simulink model "Seal"  (R2025a)
settings: Solver=FixedStepDiscrete  StartTime=0.0  StopTime=30  FixedStep=0.025  RelTol=1e-3
model workspace (MATLAB code in the model file + MAT data in the model file):
  | cmdLim = Simulink.Parameter;
  | cmdLim.Value = 15;
  | cmdLim.Description = 'Limit for controlling the maximum surface command angle.';
  | cmdLim.Min = 0;
  | cmdLim.Max = 90;
  | cmdLim.DocUnits = 'deg';
  | 
  | dispGain = Simulink.Parameter;
  | dispGain.Value = 0.75;
  | dispGain.Description = 'Gain applied to the displacement error.';
  | dispGain.Min = 0;
  | dispGain.Max = [];
  | dispGain.DocUnits = 'deg/sec/deg';
  | 
  | dispLim = Simulink.Parameter;
  | dispLim.Value = 30;
  | dispLim.Description = 'Limit for controlling the maximum commanded angle.';
  | dispLim.Min = 0;
  | dispLim.Max = 180;
  | dispLim.DocUnits = 'deg';
  | 
  | intGain = Simulink.Parameter;
  | intGain.Value = 0.5;
  | intGain.Description = 'Gain applied to the integral error.';
  | intGain.Min = 0;
  | intGain.Max = [];
  | intGain.DocUnits = 'deg/sec/deg/sec';
  | 
  | intLim = Simulink.Parameter;
  | intLim.Value = 5;
  | intLim.Description = 'Limit for controlling the maximum commanded angle.';
  | intLim.Min = 0;
  | intLim.Max = 90;
  | intLim.DocUnits = 'deg';
  | 
  | rateGain = Simulink.Parameter;
  | rateGain.Value = 2;
  | rateGain.Description = 'Gain applied to the rate error.';
  | rateGain.Min = 0;
  | rateGain.Max = [];
  | rateGain.DocUnits = 'deg/deg/sec';
  | 
  | rateLim = Simulink.Parameter;
  | rateLim.Value = 6;
  | rateLim.Description = 'Limit for controlling the maximum commanded angle.';
  | rateLim.Min = 0;
  | rateLim.Max = 180;
  | rateLim.DocUnits = 'deg/sec';
  | 
  | hdgGain = Simulink.Parameter;
  | hdgGain.Value = 0.015;
undefined symbols (not defined in the file or in its folder): CurrentCommand, KiSpeed, Kp, KpSpeed, PositionCommand, SpeedCommand
libraries: simulink x1
Description:
  | This model represents a basic roll axis autopilot with two operating
  | modes; roll attitude hold and heading hold. The mode logic for these
  | modes is external to this model.  The model architecture represents the
  | heading hold mode and basic roll attitude function as referenced models.
  | 
  | The roll attitude control function is a PID controller that uses roll
  | attitude and roll rate feedback to produce an aileron command.  The
  | input to the controller will be either a basic roll angle reference or a
  | roll command to track the desired heading.
settings Model: RequirementInfo={} %GIDa_fe9045fd_0412_4b6e_8206_617cc20e6fde  DataDictionary=SEALGenericTypes_1.sldd  FPTRunName=Active  ModifiedByFormat=The MathWorks, Inc.  Creator=The MathWorks, Inc.  LastModifiedBy=The MathWorks, Inc.
settings SolverCC: AlgebraicLoopSolver=TrustRegion
settings DataIOCC: ExternalInput=xin  SaveFormat=StructureWithTime  SaveOutput=off  SignalLogging=off  DSMLogging=off  SaveTime=off  ReturnWorkspaceOutputs=off
settings OptimizationCC: DefaultParameterBehavior=Inlined  UseDivisionForNetSlopeComputation=on  UseFloatMulNetSlope=on  InlineInvariantSignals=on  ReuseModelBlockBuffer=off  EnhancedBackFolding=on  BooleansAsBitfields=on  PassReuseOutputArgsAs=Individual arguments  ExpressionDepthLimit=2147483647.0  StateBitsets=on  DataBitsets=on  ZeroExternalMemoryAtStartup=off  ZeroInternalMemoryAtStartup=off  NoFixptDivByZeroProtection=on  EfficientFloat2IntCast=on  LifeSpan=inf  MaxStackSize=inf  EfficientTunableParamExpr=on
settings DebuggingCC: SignalRangeChecking=error  ReadBeforeWriteMsg=EnableAllAsError  WriteAfterWriteMsg=EnableAllAsError  WriteAfterReadMsg=EnableAllAsError  AlgebraicLoopMsg=error  ArtificialAlgebraicLoopMsg=error  SaveWithDisabledLinksMsg=error  SaveWithParameterizedLinksMsg=error  CheckExecutionContextPreStartOutputMsg=on  BlockPriorityViolationMsg=error  MaxConsecutiveZCsMsg=warning  SolverPrmCheckMsg=error  InheritedTsInSrcMsg=error  SingleTaskRateTransMsg=error  TasksWithSamePriorityMsg=error  SigSpecEnsureSampleTimeMsg=error  IntegerOverflowMsg=error  ParameterUnderflowMsg=error  ParameterPrecisionLossMsg=none  ParameterTunabilityLossMsg=error  UnderSpecifiedDataTypeMsg=error  UnnecessaryDatatypeConvMsg=warning  VectorMatrixConversionMsg=error  SignalLabelMismatchMsg=error  UnconnectedInputMsg=error  UnconnectedOutputMsg=error  UnconnectedLineMsg=error  SFcnCompatibilityMsg=error  UniqueDataStoreMsg=error  BusObjectLabelMismatch=error  RootOutportRequireBusObject=error  AssertControl=DisableAll  AllowSymbolicDim=off  ModelReferenceIOMismatchMessage=error  UnknownTsInhSupMsg=error  ModelReferenceDataLoggingMessage=error  ModelReferenceSymbolNameMessage=none  StateNameClashWarn=warning  StrictBusMsg=ErrorOnBusTreatedAsVector  NonBusSignalsTreatedAsBus=error  SFInvalidInputDataAccessInChartInitDiag=error  SFTransitionOutsideNaturalParentDiag=error  SFUnreachableExecutionPathDiag=error  SFUndirectedBroadcastEventsDiag=error  SFExecutionAtInitializationDiag=none  IntegerSaturationMsg=error  ArithmeticOperatorsInVariantConditions=warning
settings HardwareCC: ProdBitPerChar=16.0  ProdBitPerInt=16.0  ProdBitPerPointer=32.0  ProdBitPerSizeT=32.0  ProdBitPerPtrDiffT=32.0  ProdLargestAtomicInteger=Integer  ProdLargestAtomicFloat=None  ProdWordSize=16.0  ProdHWDeviceType=Texas Instruments->C2000  TargetHWDeviceType=32-bit Generic
settings ModelReferenceCC: EnableRefExpFcnMdlSchedulingChecks=on  ModelReferenceNumInstancesAllowed=Single  PropagateSignalLabelsOutOfModel=off
settings SFSimCC: SimUseLocalCustomCode=off  MATLABDynamicMemAlloc=off
settings SFSimCC: SimCustomHeaderCode=|
  | #include "CANServer.h"
  | #include "DeviceSetup.h"
settings SFSimCC: SimUserSources=|
  | .\ExternalCode\CANServer.c
  | .\ExternalCode\DeviceSetup.c
settings RTWCC: SystemTargetFile=ert.tlc  GenCodeOnly=on  TemplateMakefile=ert_default_tmf  PostCodeGenCommand=PrepWrapper  GenerateReport=on  RTWVerbose=off  RTWUseLocalCustomCode=off  RTWUseSimCustomCode=on  BuildConfiguration=Faster Runs  IncludeHyperlinkInReport=on  LaunchReport=on  GenerateTraceInfo=on  GenerateTraceReport=on  GenerateTraceReportSl=on  GenerateTraceReportSf=on  GenerateTraceReportEml=on  GenerateCodeMetricsReport=on  GPUComputeCapability=3.5  DLArmComputeVersion=19.05  Description=Embedded Coder
settings RTWCC: CustomHeaderCode=|
  | #include "CANServer.h"
  | #include "DeviceSetup.h"
settings RTWCC: CustomSource=|
  | .\ExternalCode\CANServer.c
  | .\ExternalCode\DeviceSetup.c
settings CodeAppCC: ForceParamTrailComments=on  IgnoreCustomStorageClasses=off  SimulinkDataObjDesc=on  CustomSymbolStrGlobalVar=rt$N$M  CustomSymbolStrType=$N$M  CustomSymbolStrFcn=$N$M$F  CustomSymbolStrMacro=$N$M  InsertBlockDesc=on  ReqsInCode=on
settings ERTTargetCC: ExtModeTransport=0.0  ExtModeStaticAlloc=off  ExtModeMexFile=ext_comm  ExtModeIntrfLevel=Level1  ERTCustomFileTemplate=example_file_process.tlc  ERTFilePackagingFormat=CompactWithDataFile  ConvertIfToSwitch=off  SuppressUnreachableDefaultCases=off  DynamicArrayContainerType=coder::array  UtilityFuncGeneration=Shared location  MultiwordLength=2048.0  GenerateSampleERTMain=on  IncludeMdlTerminateFcn=off  CombineSignalStateStructs=on  SuppressErrorStatus=on  SupportAbsoluteTime=off  SubcomponentCodeInterfacePackaging=Nonreusable function  SupportNonFinite=off  SupportComplex=off
settings ConfigComp: CovScope=ReferencedModels  CovSaveName=covdata_rollAP  CovMetricSettings=dcmtrwe  CovHTMLOptions=-sRT=1 -aTS=1 -bRG=1 -bTC=1 -hTR=1 -nFC=0 -scm=1 -bcm=1 -xEv=0  CovSaveCumulativeToWorkspaceVar=on  CovSaveSingleToWorkspaceVar=on  CovCumulativeVarName=covCumulativeData_rollAP  CovReportOnPause=off  CovExternalEMLEnable=off  CovSFcnEnable=off  DVMaxProcessTime=300.0  DVModelCoverageObjectives=MCDC  DVMaxTestCaseSteps=500.0  DVTestSuiteOptimization=Auto  DVAbsoluteTolerance=1.0e-5  DVDefectChecker=off  DVDetectActiveLogic=on  DVMaxViolationSteps=20.0  DVSaveHarnessModel=on  DVModelReferenceHarness=on  DVHarnessSource=Signal Editor  DVSaveReport=on  DVRebuildModelRepresentation=Always  DVActiveTab=0.0

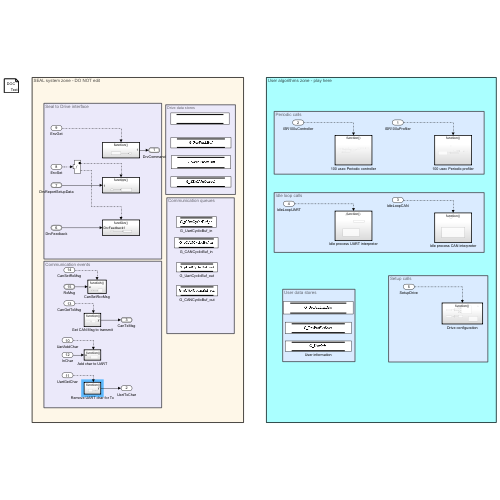
[thumbnail: Simulink's stored preview of the top-level diagram]
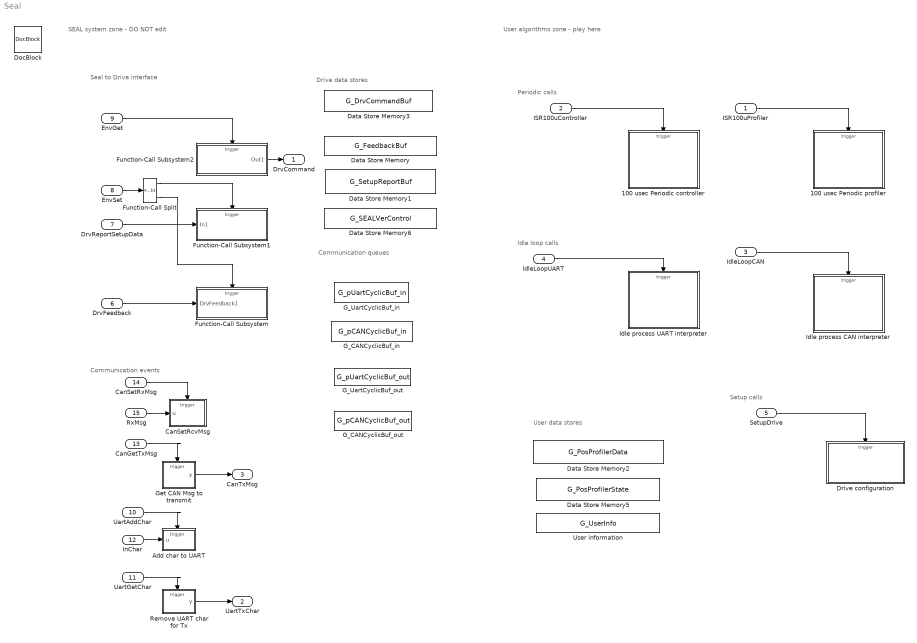
== system Seal ==
  note: User algorithms zone - play here
  note: SEAL system zone - DO NOT edit
  note: Communication queues
  note: Communication events
  note: Seal to Drive interface
  note: Setup calls
  note: Idle loop calls
  note: Periodic calls
  note: User data stores
  note: Drive data stores
  ISR100uProfiler : Inport  Priority=1  OutputFunctionCall=on
  ISR100uController : Inport  Priority=1  Port=2  OutputFunctionCall=on
  IdleLoopCAN : Inport  Priority=1  Port=3  OutputFunctionCall=on
  IdleLoopUART : Inport  Priority=1  Port=4  OutputFunctionCall=on
  SetupDrive : Inport  Priority=1  Port=5  OutputFunctionCall=on
  DrvFeedback : Inport  Port=6  OutDataTypeStr=Bus: FeedbackBuf_T  PortDimensions=1  BusOutputAsStruct=on
  DrvReportSetupData : Inport  Port=7  OutDataTypeStr=Bus: SetupReportBuf_T  PortDimensions=1  BusOutputAsStruct=on
  EnvSet : Inport  Priority=1  Port=8  OutputFunctionCall=on
  EnvGet : Inport  Priority=1  Port=9  OutputFunctionCall=on
  UartAddChar : Inport  Priority=1  Port=10  OutputFunctionCall=on
  UartGetChar : Inport  Priority=1  Port=11  OutputFunctionCall=on
  InChar : Inport  Port=12  PortDimensions=1
  CanGetTxMsg : Inport  Priority=1  Port=13  OutputFunctionCall=on
  CanSetRxMsg : Inport  Priority=1  Port=14  OutputFunctionCall=on
  RxMsg : Inport  Port=15  OutDataTypeStr=Bus: CANMessage_T  PortDimensions=1  BusOutputAsStruct=on
  100 usec Periodic controller : Subsystem  TreatAsAtomicUnit=on
  100 usec Periodic profiler : Subsystem  TreatAsAtomicUnit=on
  Add char to UART : Subsystem  TreatAsAtomicUnit=on
  CanSetRcvMsg : Subsystem  TreatAsAtomicUnit=on
  Data Store Memory : DataStoreMemory  DataStoreName=G_FeedbackBuf  WriteAfterWriteMsg=warning  VectorParams1D=off  ShowAdditionalParam=off  OutDataTypeStr=Bus: FeedbackBuf_T  StateMustResolveToSignalObject=on
  Data Store Memory1 : DataStoreMemory  DataStoreName=G_SetupReportBuf  WriteAfterWriteMsg=warning  ShowAdditionalParam=off  OutDataTypeStr=Bus: SetupReportBuf_T  StateMustResolveToSignalObject=on
  Data Store Memory2 : DataStoreMemory  DataStoreName=G_PosProfilerData  WriteAfterWriteMsg=warning  InitialValue=PosProfilerData_init  ShowAdditionalParam=off  OutDataTypeStr=Bus: PosProfilerData_T
  Data Store Memory3 : DataStoreMemory  DataStoreName=G_DrvCommandBuf  WriteAfterWriteMsg=warning  ShowAdditionalParam=off  OutDataTypeStr=Bus: DrvCommandBuf_T  StateMustResolveToSignalObject=on
  Data Store Memory5 : DataStoreMemory  DataStoreName=G_PosProfilerState  WriteAfterWriteMsg=warning  InitialValue=PosProfilerState_init  ShowAdditionalParam=off  OutDataTypeStr=Bus: PosProfilerState_T
  Data Store Memory6 : DataStoreMemory  DataStoreName=G_SEALVerControl  WriteAfterWriteMsg=warning  InitialValue=SEALVerControl_init  ShowAdditionalParam=off  OutDataTypeStr=Bus: SEALVerControl_T  StateMustResolveToSignalObject=on
  DocBlock : simulink/Model-Wide Utilities/DocBlock  DocumentType=Text
      content=|
      | These are the global variables for communication with the hosting servo drive.
      | NEVER remove them!
      | They are declared as global variables of the drive.
      | Their structure   is given in the p-coded file HostDriveInterface.p
      |
      | G_DrvCommandBuf     stores the commands to the servo drive.
      | G_SetupReportBuf    reports the setup parameters of the hosting servo drive to the SEAL application
      | FeedbackBuf         reports the feedback and sensor values to the SEAL application.
  Drive configuration : Subsystem  TreatAsAtomicUnit=on
  Function-Call Split : FunctionCallSplit  IconShape=distinctive  NumOutputPorts=2  OutputPortLayout=default
  Function-Call Subsystem : Subsystem  TreatAsAtomicUnit=on
  Function-Call Subsystem1 : Subsystem  TreatAsAtomicUnit=on
  Function-Call Subsystem2 : Subsystem  TreatAsAtomicUnit=on
  G_CANCyclicBuf_in : DataStoreMemory  DataStoreName=G_pCANCyclicBuf_in  WriteAfterWriteMsg=warning  ShowAdditionalParam=off  OutDataTypeStr=Bus: CANCyclicBuf_T  StateMustResolveToSignalObject=on
  G_CANCyclicBuf_out : DataStoreMemory  DataStoreName=G_pCANCyclicBuf_out  WriteAfterWriteMsg=warning  ShowAdditionalParam=off  OutDataTypeStr=Bus: CANCyclicBuf_T  StateMustResolveToSignalObject=on
  G_UartCyclicBuf_in : DataStoreMemory  DataStoreName=G_pUartCyclicBuf_in  WriteAfterWriteMsg=warning  ShowAdditionalParam=off  OutDataTypeStr=Bus: UartCyclicBuf_T  Dimensions=1  StateMustResolveToSignalObject=on
  G_UartCyclicBuf_out : DataStoreMemory  DataStoreName=G_pUartCyclicBuf_out  WriteAfterWriteMsg=warning  ShowAdditionalParam=off  OutDataTypeStr=Bus: UartCyclicBuf_T  StateMustResolveToSignalObject=on
  Get CAN Msg to transmit : Subsystem  TreatAsAtomicUnit=on
  Idle process CAN interpreter : Subsystem  TreatAsAtomicUnit=on
  Idle process UART interpreter : Subsystem  TreatAsAtomicUnit=on
  Remove UART char for Tx : Subsystem  TreatAsAtomicUnit=on
  User information : DataStoreMemory  DataStoreName=G_UserInfo  WriteAfterWriteMsg=warning  InitialValue=G_UserInfo_init  ShowAdditionalParam=off  OutDataTypeStr=Bus: UserInfo_T
  DrvCommand : Outport  OutDataTypeStr=Bus: DrvCommandBuf_T
  UartTxChar : Outport  Port=2  OutDataTypeStr=uint16
  CanTxMsg : Outport  Port=3  OutDataTypeStr=Bus: CANMessage_T  PortDimensions=1
  wires:
  ISR100uProfiler/1 -> 100 usec Periodic profiler/Trigger
  IdleLoopCAN/1 -> Idle process CAN interpreter/Trigger
  IdleLoopUART/1 -> Idle process UART interpreter/Trigger
  SetupDrive/1 -> Drive configuration/Trigger
  ISR100uController/1 -> 100 usec Periodic controller/Trigger
  DrvFeedback/1 -> Function-Call Subsystem/1(DrvFeedback1)
  DrvReportSetupData/1 -> Function-Call Subsystem1/1(In1)
  Function-Call Subsystem2/1(Out1) -> DrvCommand/1
  EnvSet/1 -> Function-Call Split/1
  InChar/1 -> Add char to UART/1(u)
  UartAddChar/1 -> Add char to UART/Trigger
  UartGetChar/1 -> Remove UART char for Tx/Trigger
  Remove UART char for Tx/1(y) -> UartTxChar/1
  CanGetTxMsg/1 -> Get CAN Msg to transmit/Trigger
  Get CAN Msg to transmit/1(y) -> CanTxMsg/1
  CanSetRxMsg/1 -> CanSetRcvMsg/Trigger
  RxMsg/1 -> CanSetRcvMsg/1(u)
  Function-Call Split/2 -> Function-Call Subsystem/Trigger
  Function-Call Split/1 -> Function-Call Subsystem1/Trigger
  EnvGet/1 -> Function-Call Subsystem2/Trigger

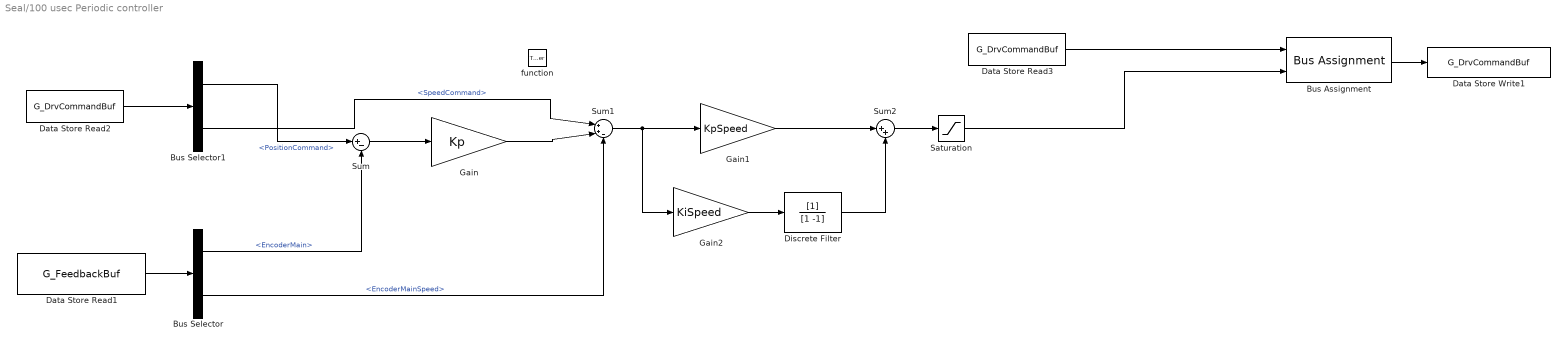
== system Seal/100 usec Periodic controller ==
  function : TriggerPort  TriggerType=function-call  VariantControl=(inherit)
  Bus Assignment : BusAssignment  AssignedSignals=CurrentCommand
  Bus Selector : BusSelector  OutputSignals=EncoderMain,EncoderMainSpeed
  Bus Selector1 : BusSelector  OutputSignals=PositionCommand,SpeedCommand
  Data Store Read1 : DataStoreRead  DataStoreName=G_FeedbackBuf  IndexOptions=Index vector (dialog)  Indices=1  OutputSizes=1
  Data Store Read2 : DataStoreRead  DataStoreName=G_DrvCommandBuf  IndexOptions=Index vector (dialog)  Indices=1  OutputSizes=1
  Data Store Read3 : DataStoreRead  DataStoreName=G_DrvCommandBuf  IndexOptions=Index vector (dialog)  Indices=1  OutputSizes=1
  Data Store Write1 : DataStoreWrite  DataStoreName=G_DrvCommandBuf  IndexOptions=Index vector (dialog)  Indices=1  OutputSizes=1
  Discrete Filter : DiscreteFilter  Denominator=[1 -1]
  Gain : Gain  Gain=Kp
  Gain1 : Gain  Gain=KpSpeed
  Gain2 : Gain  Gain=KiSpeed
  Saturation : Saturate
  Sum : Sum  Inputs=|+-
  Sum1 : Sum  Inputs=|++-
  Sum2 : Sum  Inputs=|++
  wires:
  Data Store Read3/1 -> Bus Assignment/1
  Bus Assignment/1 -> Data Store Write1/1
  Data Store Read1/1 -> Bus Selector/1
  Bus Selector/1 -> Sum/2  "<EncoderMain>"
  Data Store Read2/1 -> Bus Selector1/1
  Bus Selector1/1 -> Sum/1  "<PositionCommand>"
  Sum/1 -> Gain/1
  Gain/1 -> Sum1/2
  Bus Selector1/2 -> Sum1/1  "<SpeedCommand>"
  Bus Selector/2 -> Sum1/3  "<EncoderMainSpeed>"
  Sum1/1 -> Gain2/1, Gain1/1
  Gain2/1 -> Discrete Filter/1
  Gain1/1 -> Sum2/1
  Discrete Filter/1 -> Sum2/2
  Sum2/1 -> Saturation/1
  Saturation/1 -> Bus Assignment/2

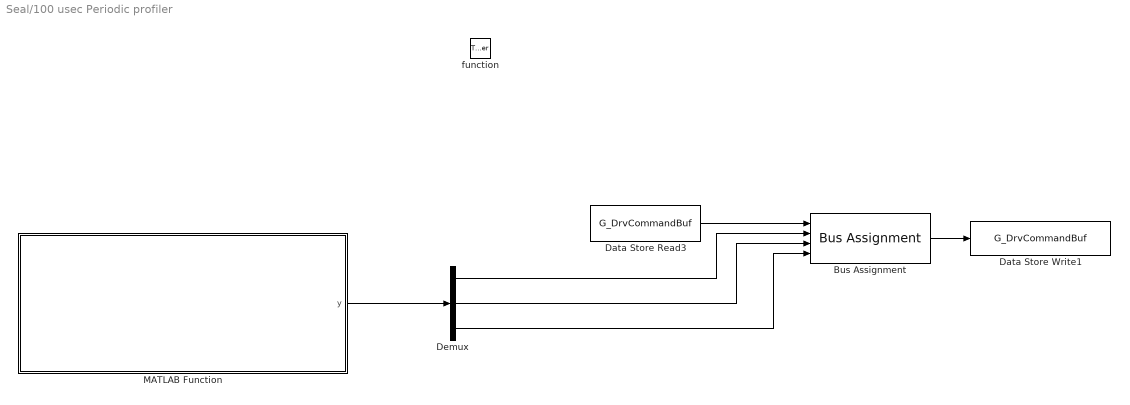
== system Seal/100 usec Periodic profiler ==
  function : TriggerPort  TriggerType=function-call  VariantControl=(inherit)
  Bus Assignment : BusAssignment  AssignedSignals=PositionCommand,SpeedCommand,CurrentCommand
  Data Store Read3 : DataStoreRead  DataStoreName=G_DrvCommandBuf  IndexOptions=Index vector (dialog)  Indices=1  OutputSizes=1
  Data Store Write1 : DataStoreWrite  DataStoreName=G_DrvCommandBuf  IndexOptions=Index vector (dialog)  Indices=1  OutputSizes=1
  Demux : Demux  Outputs=3
  MATLAB Function : MATLAB Function  TreatAsAtomicUnit=on
  wires:
  Data Store Read3/1 -> Bus Assignment/1
  MATLAB Function/1(y) -> Demux/1
  Demux/1 -> Bus Assignment/2
  Demux/2 -> Bus Assignment/3
  Demux/3 -> Bus Assignment/4
  Bus Assignment/1 -> Data Store Write1/1

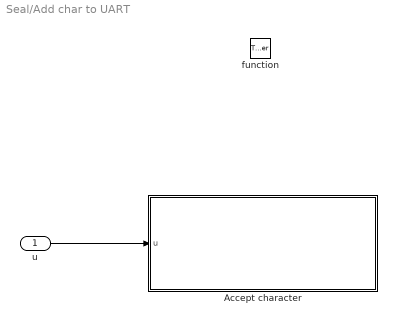
== system Seal/Add char to UART ==
  u : Inport  OutDataTypeStr=uint16  PortDimensions=1
  function : TriggerPort  TriggerType=function-call  VariantControl=(inherit)
  Accept character : MATLAB Function  TreatAsAtomicUnit=on
  wires:
  u/1 -> Accept character/1(u)

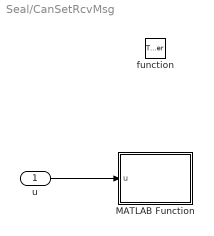
== system Seal/CanSetRcvMsg ==
  u : Inport  OutDataTypeStr=Bus: CANMessage_T
  function : TriggerPort  TriggerType=function-call  VariantControl=(inherit)
  MATLAB Function : MATLAB Function  TreatAsAtomicUnit=on
  wires:
  u/1 -> MATLAB Function/1(u)

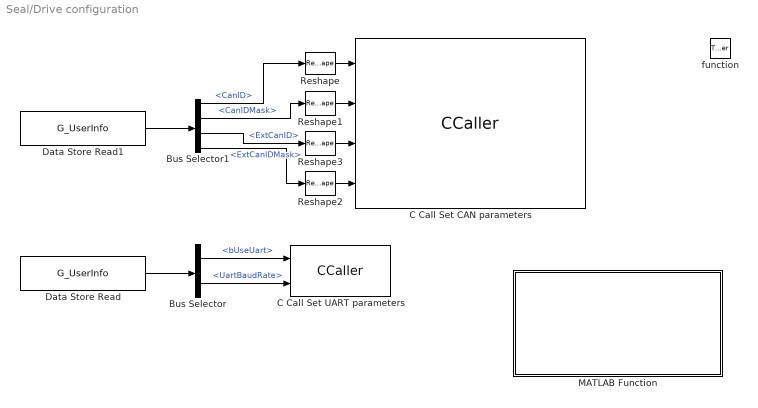
== system Seal/Drive configuration ==
  function : TriggerPort  TriggerType=function-call  VariantControl=(inherit)
  Bus Selector : BusSelector  OutputSignals=bUseUart,UartBaudRate
  Bus Selector1 : BusSelector  OutputSignals=CanID,CanIDMask,ExtCanID,ExtCanIDMask
  C Call Set CAN parameters : CCaller  FunctionName=SetCanParameters  PortSpecificationStruct="%)30     .    6 <   8    (     @         %    \"     0    !     0         %  0 \"0    $    _    07)G3F%M90  4&]R=$YA;64 4V-O<&4     26YD97@     5'EP90      4VEZ90      27-';&]B86P   X    X    !@    @    $          4    (     0    4    !         !     %    0V%N240    .    .     8    (    !          %    \"     $    %     0         0    !0   $-A;DE$    #@   #@    &    \"     0         !0    @    !   ...(+2149 chars)"
  C Call Set UART parameters : CCaller  FunctionName=SetUartParameters  PortSpecificationStruct="%)30     .    V ,   8    (     @         %    \"     (    !     0         %  0 \"0    $    _    07)G3F%M90  4&]R=$YA;64 4V-O<&4     26YD97@     5'EP90      4VEZ90      27-';&]B86P   X    X    !@    @    $          4    (     0    <    !         !     '    =7-E56%R=  .    .     8    (    !          %    \"     $    '     0         0    !P   '5S955A<G0 #@   #@    &    \"     0         !0    @    !    !0    $         $     4   !);G!U=     X    X    !@    @    &          4    (     0    $    !          D    (               .    .     8    (    !          %    \"     $    &     0         0    !@   '5I;G0Q-@  #@   #     &    \"     0         !0    @    !     0    $         $  ! #$    .    ,     8    (    \"0(        %    \"     $    !     0         \"  $       X    X    !@    @    $          4    (     0    @    !         !     (    8F%U9%)A=&4.    .     8    (    !          %    \"     $    (     0         0    \"    &)A=612871E#@   #@    &    \"     0         !0    @    !    !0    $         $     4   !);G!U=     X    X    !@    @    &          4    (     0    $    !          D    (            \\#\\.    .     8    (    !          %    \"     $    &     0         0    !@   '5I;G0S,@  #@   #     &    \"     0         !0    @    !     0    $         $  ! #$    .    ,     8    (    \"0(        %    \"     $    !     0         \"  $"
  Data Store Read : DataStoreRead  DataStoreName=G_UserInfo  IndexOptions=Index vector (dialog)  Indices=1  OutputSizes=1
  Data Store Read1 : DataStoreRead  DataStoreName=G_UserInfo  IndexOptions=Index vector (dialog)  Indices=1  OutputSizes=1
  MATLAB Function : MATLAB Function  TreatAsAtomicUnit=on
  Reshape{,1..3} (4 alike) : Reshape
  wires:
  Data Store Read/1 -> Bus Selector/1
  Bus Selector/1 -> C Call Set UART parameters/1  "<bUseUart>"
  Bus Selector/2 -> C Call Set UART parameters/2  "<UartBaudRate>"
  Data Store Read1/1 -> Bus Selector1/1
  Bus Selector1/1 -> Reshape/1  "<CanID>"
  Bus Selector1/2 -> Reshape1/1  "<CanIDMask>"
  Bus Selector1/4 -> Reshape2/1  "<ExtCanIDMask>"
  Reshape/1 -> C Call Set CAN parameters/1
  Reshape1/1 -> C Call Set CAN parameters/2
  Reshape2/1 -> C Call Set CAN parameters/4
  Bus Selector1/3 -> Reshape3/1  "<ExtCanID>"
  Reshape3/1 -> C Call Set CAN parameters/3

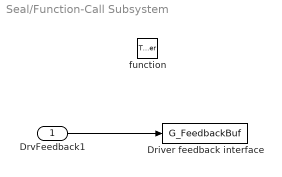
== system Seal/Function-Call Subsystem ==
  DrvFeedback1 : Inport
  function : TriggerPort  TriggerType=function-call  VariantControl=(inherit)
  Driver feedback interface : DataStoreWrite  DataStoreName=G_FeedbackBuf  IndexOptions=Index vector (dialog)  Indices=1  OutputSizes=1
  wires:
  DrvFeedback1/1 -> Driver feedback interface/1

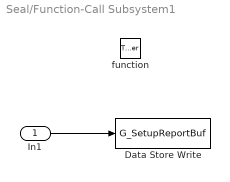
== system Seal/Function-Call Subsystem1 ==
  In1 : Inport
  function : TriggerPort  TriggerType=function-call  VariantControl=(inherit)
  Data Store Write : DataStoreWrite  DataStoreName=G_SetupReportBuf  IndexOptions=Index vector (dialog)  Indices=1  OutputSizes=1
  wires:
  In1/1 -> Data Store Write/1

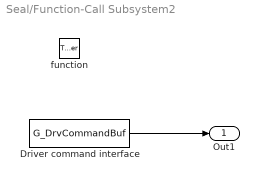
== system Seal/Function-Call Subsystem2 ==
  function : TriggerPort  TriggerType=function-call  VariantControl=(inherit)
  Driver command interface : DataStoreRead  DataStoreName=G_DrvCommandBuf  IndexOptions=Index vector (dialog)  Indices=1  OutputSizes=1
  Out1 : Outport
  wires:
  Driver command interface/1 -> Out1/1

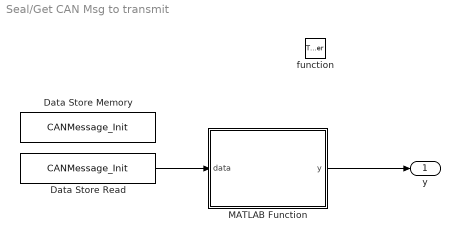
== system Seal/Get CAN Msg to transmit ==
  function : TriggerPort  TriggerType=function-call  VariantControl=(inherit)
  Data Store Memory : DataStoreMemory  DataStoreName=CANMessage_Init  WriteAfterWriteMsg=warning  ShowAdditionalParam=off  OutDataTypeStr=Bus: CANMessage_T
  Data Store Read : DataStoreRead  DataStoreName=CANMessage_Init  IndexOptions=Index vector (dialog)  Indices=1  OutputSizes=1
  MATLAB Function : MATLAB Function  TreatAsAtomicUnit=on
  y : Outport
  wires:
  MATLAB Function/1(y) -> y/1
  Data Store Read/1 -> MATLAB Function/1(data)

== system Seal/Idle process CAN interpreter ==
  function : TriggerPort  TriggerType=function-call  VariantControl=(inherit)
  CAN message response : MATLAB Function  TreatAsAtomicUnit=on

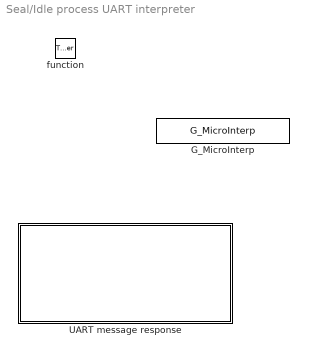
== system Seal/Idle process UART interpreter ==
  function : TriggerPort  TriggerType=function-call  VariantControl=(inherit)
  G_MicroInterp : DataStoreMemory  DataStoreName=G_MicroInterp  WriteAfterWriteMsg=warning  ShowAdditionalParam=off  OutDataTypeStr=Bus: MicroInterp_T  StateMustResolveToSignalObject=on
      settings: LockScale=on
  UART message response : MATLAB Function  TreatAsAtomicUnit=on

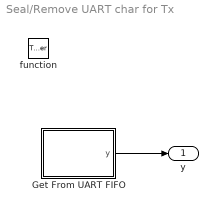
== system Seal/Remove UART char for Tx ==
  function : TriggerPort  TriggerType=function-call  VariantControl=(inherit)
  Get From UART FIFO : MATLAB Function  TreatAsAtomicUnit=on
  y : Outport
  wires:
  Get From UART FIFO/1(y) -> y/1

== matlab function Seal/Idle process CAN interpreter/CAN message response ==
  data: G_pCANCyclicBuf_in data_store_memory; G_pCANCyclicBuf_out data_store_memory
function OutBuf



global G_pCANCyclicBuf_in  
global G_pCANCyclicBuf_out  

if (G_pCANCyclicBuf_in.PutCounter == G_pCANCyclicBuf_in.FetchCounter ) 
    return ; 
end

for cnt = 1:3 
% The CAN queues count like C (zero based), yet the code here is matlab (1
% based) so we have to increment the counters to be valid Matlab indices
    nfetch  = bitand( G_pCANCyclicBuf_in.FetchCounter ,63 ) + 1; 
    nput    = bitand( G_pCANCyclicBuf_out.PutCounter  , 63) + 1 ; 
    nextput = bitand( nput + 1 , 63)  ;  
    if ( nextput == G_pCANCyclicBuf_out.FetchCounter) 
        break ; % Output queue is full 
    end 

    nmsgGet     = nfetch * 2 - 1 ; 
    nmsgPut     = nput  * 2 -  1 ; 
    nextmsg     = G_pCANCyclicBuf_in.CANQueue([nmsgGet,nmsgGet+1]) ;

    nextid      = G_pCANCyclicBuf_in.CANID(nfetch) ; 
    nextattrib  = G_pCANCyclicBuf_in.DLenAndAttrib(nfetch) ; 

    % Idiotic interpreter - just return what it got 
    G_pCANCyclicBuf_out.CANQueue([nmsgPut,nmsgPut+1]) = nextmsg; 
    G_pCANCyclicBuf_out.CANID(nput) = nextid ; 
    G_pCANCyclicBuf_out.DLenAndAttrib(nput) = nextattrib ;

    % Update TX and RX counters
    G_pCANCyclicBuf_out.PutCounter  = nextput ;
    G_pCANCyclicBuf_in.FetchCounter = bitand( nfetch + 1  , 63) ; 

    if (G_pCANCyclicBuf_in.PutCounter == G_pCANCyclicBuf_in.FetchCounter ) 
        break ; 
    end
end


end
% celems(1) = SetBusElement('PutCounter','uint16',"The place in the CANQueue where the next message is to be put" ) ; 
% celems(2) = SetBusElement('FetchCounter','uint16',"The location in the CANQueue of the next message to read" ) ; 
% celems(3) = SetBusElement('CANError','uint16',"CAN error" ) ; 
% celems(4) = SetBusElement('CANQueue','uint32',"Software Queue for incoming UART characters" ,[64,2]) ; 
% celems(5) = SetBusElement('TxFetchCounter','uint16',"The location in the CANQueue of the next message to transmit" ) ; 
% celems(6) = SetBusElement('CANID','uint32',"Can ID, 11 or 29bit" ,[64,1]) ; 
% celems(7) = SetBusElement('DLenAndAttrib','uint16',"Data length and attributes" ,[64,1]) ;

== matlab function Seal/100 usec Periodic profiler/MATLAB Function ==
  data: y output double size=[3,1]; G_PosProfilerState data_store_memory; G_PosProfilerData data_store_memory; G_SetupReportBuf data_store_memory
function y  = fcn

global G_PosProfilerState
global G_PosProfilerData
global G_SetupReportBuf

Ts = double( G_PosProfilerData.Ts) ; 
% Copy state for use 

y = zeros(3,1) ; 
if ( G_PosProfilerData.ProfileDataOk == 0 )
    speed =  max( abs(G_PosProfilerState.Speed)-Ts*G_SetupReportBuf.AbsoluteAccelerationLimit , 0 ) * sign(G_PosProfilerState.Speed); 
    pos    = G_PosProfilerState.Position + ( speed + G_PosProfilerState.Speed ) * Ts* 0.5  ;  
    NewFiltState4 = double(pos) ; 
    NewFiltState3 = double(pos) ; 
    NewFiltState2 = double(pos) ; 
    NewFiltState1 = double(pos) ; 
else  
    % Advance profiler 
    Delta = G_PosProfilerData.PositionTarget - G_PosProfilerState.Position - G_PosProfilerState.Speed * Ts * 0.5  ; 
    Direction = 1 ; 
    if ( Delta < 0  )
        Direction = -1 ; 
        Delta = -Delta ;
        speed  = -G_PosProfilerState.Speed ; 
    else
        speed  = G_PosProfilerState.Speed ; 
    end 
        
    desiredSpeed = sqrt(Delta * 2 * G_PosProfilerData.ProfileDeceleration ) ; 
    if ( speed < desiredSpeed  ) 
        speed = min ([speed +Ts * G_PosProfilerData.ProfileDeceleration , G_PosProfilerData.ProfileSpeed  , desiredSpeed] ) ; 
    else
        speed = max(desiredSpeed , speed - Ts * G_PosProfilerData.ProfileDeceleration * 1.02   ) ;  
    end
    speed = speed * Direction ; 

    % tf(2 ,conv([1,2],[1,1.71,1]) )
    pos    = G_PosProfilerState.Position + ( speed +  G_PosProfilerState.Speed ) * Ts* 0.5  ;  
    NewFiltState4 = G_PosProfilerState.FiltState(3) ; 
    NewFiltState3 = G_PosProfilerState.FiltState(2) ; 
    NewFiltState2 = G_PosProfilerState.FiltState(1) ;
    NewFiltState1 = -(G_PosProfilerState.FiltState(1) * G_PosProfilerData.ProfileFilterDen(2) + ...
        G_PosProfilerState.FiltState(2) * G_PosProfilerData.ProfileFilterDen(3) + ...
        G_PosProfilerState.FiltState(3) * G_PosProfilerData.ProfileFilterDen(4)) + double(pos) * G_PosProfilerData.ProfileFilterNum ; 

end
G_PosProfilerState.Position =  double(pos)   ; 
G_PosProfilerState.Speed    =  double(speed) ; 
y = [NewFiltState1 ; (NewFiltState1-G_PosProfilerState.FiltState(1))/ max(Ts,1e-5); 0 ] ;  
G_PosProfilerState.FiltState = [NewFiltState1;NewFiltState2;NewFiltState3;NewFiltState4] ;

end

== matlab function Seal/Idle process UART interpreter/UART message response ==
  data: G_pUartCyclicBuf_in data_store_memory; G_pUartCyclicBuf_out data_store_memory; G_MicroInterp data_store_memory
function UARTHandler()

%global   
global G_MicroInterp      
global G_pUartCyclicBuf_in

for cnt = 1:10 
% The CAN queues count like C (zero based), yet the code here is matlab (1
% based) so we have to increment the counters to be valid Matlab indices
    if (G_pUartCyclicBuf_in.PutCounter == G_pUartCyclicBuf_in.FetchCounter ) 
        return ; 
    end

    nmsgGet     = bitand( G_pUartCyclicBuf_in.FetchCounter, 255) ; 
    nextfetch   = bitand( nmsgGet + 1, 255 ); 
    nextmsg     = G_pUartCyclicBuf_in.UARTQueue(nmsgGet + 1 ) ;
    G_pUartCyclicBuf_in.FetchCounter = nextfetch ; 

    if G_pUartCyclicBuf_in.UartError 
        G_pUartCyclicBuf_in.UartError = uint16(0) ; 
        G_MicroInterp.InterpretError = uint16(3) ; 
        continue ; 
    end

    StringFormatter(nextmsg) ; 
    if ( G_MicroInterp.NewString )
        StringMicroSplitter() ;  
        if G_MicroInterp.InterpretError== uint16(0) 
            MicroInterpret() ; 
            FormatInterpreterResponse() ;
            SendTxResponse();
        end
    end
end
end

function FormatInterpreterResponse() 
    global G_MicroInterp 
    if ( G_MicroInterp.InterpretError) 
        
            
        G_MicroInterp.TempString(1) = 'E' ; 
        G_MicroInterp.TempString(2) = 'R' ; 
        G_MicroInterp.TempString(3) = 'R' ; 
        G_MicroInterp.TempString(4) = 'O' ; 
        G_MicroInterp.TempString(5) = 'R' ; 
        G_MicroInterp.TempString(6) = ':' ; 
        G_MicroInterp.cnt = uint16(6) ; 
        errnum = G_MicroInterp.InterpretError ; 
        while ( errnum )
            G_MicroInterp.cnt = G_MicroInterp.cnt + uint16(1) ;
            nextdigit = uint16(mod( errnum , 10 )) ; 
            G_MicroInterp.TempString(G_MicroInterp.cnt) = nextdigit + uint16('0') ; 
            errnum = errnum - nextdigit ;
        end
    end

    if ( G_MicroInterp.IsGetFunc) 
        n = fix(log10(G_MicroInterp.Argument)) ; 
        SciExp = int16(0) ; 
        SciNotation = 0 ; 
        argout = G_MicroInterp.Argument  ;
        if n > 8 || n < -8   
            nafterPeriod = 8 - n  ; 
        else
            nafterPeriod = 6   ; 
            SciNotation  = 1   ; 
            SciExp = int16(n) ; 
            argout = argout * 10^(-n) ; 
            %n = 1 ; 
        end

        m = fix(argout) ; 
        while ( m )
            G_MicroInterp.cnt = G_MicroInterp.cnt + 1 ;
            nextdigit = uint16(mod( m , 10 )) ; 
            G_MicroInterp.TempString(G_MicroInterp.cnt) = nextdigit + uint16('0') ; 
            m = m - double(nextdigit) ;
        end
        if nafterPeriod > 0 
            G_MicroInterp.cnt = G_MicroInterp.cnt + 1 ;
            G_MicroInterp.TempString(G_MicroInterp.cnt) = '.' ; 
            m = fix( (argout-m) * 10^(nafterPeriod)) ; 
            while ( m )
                G_MicroInterp.cnt = G_MicroInterp.cnt + 1 ;
                nextdigit = uint16(mod( m , 10 )) ; 
                G_MicroInterp.TempString(G_MicroInterp.cnt) = nextdigit + uint16('0') ; 
                m = m - double(nextdigit) ;
            end                
        end
        if SciNotation && SciExp 
            G_MicroInterp.cnt = G_MicroInterp.cnt + 1 ;
            G_MicroInterp.TempString(G_MicroInterp.cnt) = 'E' ; 
            if ( SciExp < 0 )

                G_MicroInterp.cnt = G_MicroInterp.cnt + 1 ;
                G_MicroInterp.TempString(G_MicroInterp.cnt) = '-' ; 
                SciExp = -SciExp ; 
            end
            while ( SciExp )
                G_MicroInterp.cnt = G_MicroInterp.cnt + 1 ;
                nextdigit = uint16(mod( SciExp , 10 )) ; 
                G_MicroInterp.TempString(G_MicroInterp.cnt) = nextdigit + uint16('0') ; 
                SciExp = SciExp - int16(nextdigit) ;
            end                
        end

    end
end


function SendTxResponse()
% Transmit text to a cyclic buffer
    % Return interpreter response 
    global G_pUartCyclicBuf_out  
    global G_MicroInterp      
    for txcnt = 1 : G_MicroInterp.cnt
        nput    = bitand( G_pUartCyclicBuf_out.PutCounter  , 255)  ; 
        nextput = bitand( nput + 1 , 255)  ;  
        if ( nextput == G_pUartCyclicBuf_out.FetchCounter) 
            break ; % Output queue is full 
        end 
        G_pUartCyclicBuf_out.UARTQueue( nput+1) = G_MicroInterp.TempString(txcnt) ; 
    
        % Update TX counter
        G_pUartCyclicBuf_out.PutCounter  = nextput ;
    end
end

function MicroInterpret() 
    global G_MicroInterp      
    switch (G_MicroInterp.MnemonicIndex) 
        case 390 % PA 
            if ( G_MicroInterp.IsGetFunc )
                G_MicroInterp.Argument = GetPositionTarget() ; 
            else
                G_MicroInterp.InterpretError = SetPositionTarget(G_MicroInterp.Argument) ;  
            end
        otherwise
             G_MicroInterp.InterpretError = uint16(22); 

    end
end

function  StringFormatter(c) 

    arguments (Input)
        c uint16 
    end

    global G_MicroInterp      
    
    if ( c == ';' )
        G_MicroInterp.NewString = G_MicroInterp.cnt ; 
        return    ; 
    end
    if G_MicroInterp.NewString 
        G_MicroInterp.cnt = uint16(0) ; 
        G_MicroInterp.InterpretError = uint16(0); 
    end 

    if G_MicroInterp.InterpretError  
        return 
    end

    if ( c <= 'z' && c >= 'a')
        c = c + uint16('A') - uint16('a')   ; 
    end

    if ( c >= 9 && c <= 13) || (c == 32) || (c=='+')
        return ; %  Whitespace - ignore 
    end

    if ( G_MicroInterp.cnt >= 64 )
        G_MicroInterp.InterpretError = uint16(2) ; 
    end

    if ( c <= 'Z' && c >= 'A') || ( c <= '9' && c >= '0') || (c=='-') || (c=='=')
          G_MicroInterp.TempString(G_MicroInterp.cnt+1)  ; 
          G_MicroInterp.cnt = G_MicroInterp.cnt+1 ;
    else
        G_MicroInterp.InterpretError =  uint16(1) ; 
    end

end


function StringMicroSplitter() 
    global G_MicroInterp      
    G_MicroInterp.NewString = uint16(0) ;
    if (G_MicroInterp.cnt < 2 ) 
        return ; 
    end
    if  (G_MicroInterp.TempString(1) < 'A') || (G_MicroInterp.TempString(1) > 'Z') || ...
            (G_MicroInterp.TempString(2) < 'A') || (G_MicroInterp.TempString(2) > 'Z')  
        G_MicroInterp.InterpretError = uint16(10);  
        return ; 
    end
    G_MicroInterp.IsGetFunc  = uint16(1) ; 
    G_MicroInterp.ArrayIndex = uint16(1) ; 
    
    G_MicroInterp.MnemonicIndex = G_MicroInterp.TempString(1) * 26 + G_MicroInterp.TempString(2)  ; 
    
    % Case of scalar GET mnemonic
    if (G_MicroInterp.cnt <= 2 ) 
        return ; 
    end
    
    start = uint16(3) ; 
    if ( G_MicroInterp.TempString(3) =='[')
        gotArrayIndex = uint16(0) ; 
        G_MicroInterp.ArrayIndex = uint16(0) ; 
        for cnt = uint16(4):G_MicroInterp.cnt
            if ( G_MicroInterp.TempString(cnt) == ']')
                if ( G_MicroInterp.ArrayIndex  == 0 ) 
                    G_MicroInterp.InterpretError = uint16(11);  
                    return ; 
                end
                start = cnt + uint16(1) ; 
                gotArrayIndex = uint16(1) ; 
            else
                c = bitand(G_MicroInterp.TempString(cnt), 255 ) ; 
                if ( c < '0' || c > '9')
                    G_MicroInterp.InterpretError =  uint16(12)   ;  
                    return ; 
                end
                G_MicroInterp.ArrayIndex = bitand(G_MicroInterp.ArrayIndex ,31) * 10 + c - uint16('0') ; 
            end
        end
        if ( gotArrayIndex == 0 )
            G_MicroInterp.InterpretError = uint16(14)   ; 
            return ; 
        end
    end

    % Case of vector GET mnemonic
    if (G_MicroInterp.cnt < start ) 
        return ; 
    end
    
    if ~( G_MicroInterp.TempString(start) == '=')
        G_MicroInterp.InterpretError = uint16(15)  ;  
        return ; 
    end
    
    start = start + uint16(1) ;
    Mantissa = 0  ; 
    Exp = uint16(0) ; 
    sgnMant = int16(1) ; 
    sgnExp = int16(1) ; 
    isExp = uint16(0) ; 
    if (G_MicroInterp.cnt < start ) 
        G_MicroInterp.InterpretError = uint16(16)  ;  
        return ; 
    end
    if (G_MicroInterp.TempString(start) == '-')
        sgnMant = int16(-1) ; 
        start = start + uint16(1) ; 
        if (G_MicroInterp.cnt < start ) 
            G_MicroInterp.InterpretError = uint16(17)  ;  
            return ; 
        end
    end

    cnt = start ; 
    WasPeriod = uint16(0); 
    PeriodPos = uint16(0) ; 
    while ( cnt <= G_MicroInterp.cnt) 
        c = bitand(G_MicroInterp.TempString(cnt),255) ;  
        if ( isExp == 0 )
            if ( c >= '0' && c <= '9')
                Mantissa = Mantissa * 10 + double(c)  ; 
                cnt = cnt + uint16(1) ;
                if ( WasPeriod) 
                    PeriodPos = PeriodPos + uint16(1) ;
                end
            else
                if ( c == '.')
                    WasPeriod = uint16(1) ; 
                else
                    if ( c == 'E' )
                        cnt = cnt+ 1 ; 
                        isExp = uint16(1) ;
                        if cnt > G_MicroInterp.cnt
                            G_MicroInterp.InterpretError = uint16(19)  ;  
                            return ; 
                        end
                        if (G_MicroInterp.TempString(cnt) == '-' )
                            sgnExp = int16(-1) ; 
                            cnt = cnt+ uint16(1) ;
                            if cnt > G_MicroInterp.cnt
                                G_MicroInterp.InterpretError = uint16(20)  ;  
                                return ; 
                            end
                        end
                    else
                        G_MicroInterp.InterpretError = uint16(18)  ;  
                        return ; 
                    end
                end
            end
        else
            if ( c >= '0' && c <= '9')
                Exp = bitand(Exp,511) * 10 + c  ; 
                cnt = cnt + 1 ;
            else
                G_MicroInterp.InterpretError = uint16(21)  ;  
                return ;                 
            end
        end
        
    end
    if WasPeriod  
         Mantissa = Mantissa / double(10^single(PeriodPos)) ; 
    end
    G_MicroInterp.Argument = Mantissa * double(sgnMant) ; 
    if isExp
        G_MicroInterp.Argument = G_MicroInterp.Argument * double(10^(single(sgnExp)*single(Exp)) ) ; 
    end

end


function value = GetPositionTarget() 
value = 0 ; 
end

function errcode = SetPositionTarget(pa) 
errcode = uint16(0) ; 
end



% celems(1) = SetBusElement('PutCounter','uint16',"The place in the UARTQueue where the next message is to be put" ) ; 
% celems(2) = SetBusElement('FetchCounter','uint16',"The location in the UARTQueue of the next message to read" ) ; 
% celems(3) = SetBusElement('CANError','uint16',"CAN error" ) ; 
% celems(4) = SetBusElement('UARTQueue','uint32',"Software Queue for incoming UART characters" ,[64,2]) ; 
% celems(5) = SetBusElement('TxFetchCounter','uint16',"The location in the UARTQueue of the next message to transmit" ) ; 
% celems(6) = SetBusElement('CANID','uint32',"Can ID, 11 or 29bit" ,[64,1]) ; 
% celems(7) = SetBusElement('DLenAndAttrib','uint16',"Data length and attributes" ,[64,1]) ;

== matlab function Seal/Drive configuration/MATLAB Function ==
function SealSetup() 

global G_UserInfo

% Object Initialization code 
 SetObject2Drive( uint16(hex2dec('60f0')), uint16(1)  , single(150000) ,VarDataTypes.T_uint32) ; 

% Get object from file 
% G_UserInfo.junk1 = single( GetObjectFromDrive( uint16(hex2dec('60f0')), uint16(1) , VarDataTypes.T_uint32) ) ; 

end


function retCode = SetObject2Drive( Index, subIndex  ,value  , datatype ) 
    retCode = int32(0); 
    coder.ceval('SetObject2Drive', uint16(Index), uint16(subIndex), double(value) , uint16(datatype) ,coder.ref(retCode));
end

function [value,retCode] = GetObjectFromDrive( Index, subIndex , datatype) 
    retCode = int32(0); 
    value   = double(0) ; 
    coder.ceval('GetObjectFromDrive', uint16(Index), uint16(subIndex), uint16(datatype) , coder.ref(value), coder.ref(retCode));
end

== matlab function Seal/Add char to UART/Accept character ==
  data: u input; G_pUartCyclicBuf_in data_store_memory
function ReceiveUartChar(u)

global G_pUartCyclicBuf_in

next = uint16(bitand(G_pUartCyclicBuf_in.PutCounter,255)+ 1) ; 
if ( next == G_pUartCyclicBuf_in.FetchCounter )
    G_pUartCyclicBuf_in.UartError = uint16(1) ; 
    return ; 
end
G_pUartCyclicBuf_in.UARTQueue(G_pUartCyclicBuf_in.PutCounter)  = u ; 
G_pUartCyclicBuf_in.PutCounter = next ;

== matlab function Seal/Remove UART char for Tx/Get From UART FIFO ==
  data: y output; G_pUartCyclicBuf_out data_store_memory
function y = GetFromUartFifo
global G_pUartCyclicBuf_out 
y = G_pUartCyclicBuf_out ; 
nchars = mod( y.PutCounter - y.FetchCounter, 256 ) ; 
if ( y.PutCounter >= y.FetchCounter)
    y.UARTQueue(1:nchars) = y.UARTQueue(y.FetchCounter:y.FetchCounter+nchars-1) ; 
else
    nrem = 256 - y.FetchCounter + 1  ; 
    y.UARTQueue(1:nrem) = y.UARTQueue(y.FetchCounter:256) ;   
    if ( y.PutCounter > 1 ) 
        y.UARTQueue(nrem+1:nchars)  = y.UARTQueue(1:y.PutCounter-1) ;     
    end
end
y.PutCounter = mod( nchars + 1 , 256) ; 
y.FetchCounter = 1 ; 


% y = uint16([0;0]) ; 
% nchars = mod( G_pUartCyclicBuf_out.PutCounter - G_pUartCyclicBuf_out.FetchCounter, 256 ) ; 
% nextchar = 0 ; 
% if nchars ~= 0 
%     next = uint16(bitand ( G_pUartCyclicBuf_out.FetchCounter, 255) + 1) ; 
%     nextchar = G_pUartCyclicBuf_out.UARTQueue(next) ; 
%     G_pUartCyclicBuf_out.FetchCounter = next ;  
% end
% y(1) = uint16(nextchar) ; 
% y(2) = uint16(nchars) ;

== matlab function Seal/Get CAN Msg to transmit/MATLAB Function ==
  data: y output Bus: CANMessage_T size=1; G_pCANCyclicBuf_out data_store_memory; data input
function y = CanOutTx( data)

global G_pCANCyclicBuf_out 

y = data ; 
if ~(G_pCANCyclicBuf_out.PutCounter == G_pCANCyclicBuf_out.FetchCounter)
    next = uint16(bitand ( G_pCANCyclicBuf_out.FetchCounter, 255) + 1) ; 
    y.CANID = G_pCANCyclicBuf_out.CANID(next) ; 
    y.DataLen = G_pCANCyclicBuf_out.DLenAndAttrib(next) ; 
    y.MsgData(1) =  G_pCANCyclicBuf_out.CANQueue(next*2-1) ; 
    y.MsgData(2) =  G_pCANCyclicBuf_out.CANQueue(next*2) ; 
    y.CANTxCnt = mod( G_pCANCyclicBuf_out.FetchCounter - G_pCANCyclicBuf_out.PutCounter, 64  ) ; 
    G_pCANCyclicBuf_out.FetchCounter = next ;  
end

== matlab function Seal/CanSetRcvMsg/MATLAB Function ==
  data: u input Bus: CANMessage_T size=1; G_pCANCyclicBuf_in data_store_memory
function RcvCanMsg(u)
global G_pCANCyclicBuf_in 

next = bitand(G_pCANCyclicBuf_in.PutCounter, 63) + 1 ; 
if ( next == G_pCANCyclicBuf_in.FetchCounter)
    return ; 
end

G_pCANCyclicBuf_in.CANID(next) = u.CANID ; 
G_pCANCyclicBuf_in.CANQueue(next*2-1:next*2) = u.MsgData(1:2) ; 
G_pCANCyclicBuf_in.DLenAndAttrib(next) = u.DataLen ; 

G_pCANCyclicBuf_in.PutCounter = next ;
